simulink library "whatevs"  (R2019a)
settings: Solver=VariableStepAuto  StartTime=0.0  StopTime=10.0  RelTol=1e-3
settings Model: Creator=agmotes  LastModifiedBy=agmotes

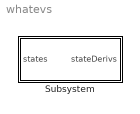
== system whatevs ==
  Subsystem : Subsystem

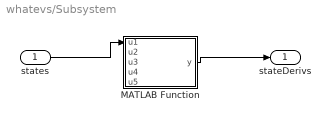
== system whatevs/Subsystem ==
  states : Inport
  MATLAB Function : MATLAB Function  TreatAsAtomicUnit=on
  stateDerivs : Outport
  wires:
  states/1 -> MATLAB Function/1(u1)
  MATLAB Function/1(y) -> stateDerivs/1

== matlab function whatevs/Subsystem/MATLAB Function ==
  data: u1 input; y output; u2 input; u3 input; u4 input; u5 input
function y = fcn(u1,u2,u3,u4,u5)
    
y = u;
